simulink model "agv_mechanical_plant"  (R2026a)
settings: Solver=VariableStepAuto  StopTime=cfg.simulation.stop_time
undefined symbols (not defined in the file): cfg
settings Model: Creator=YASHRK  LastModifiedBy=YASHRK

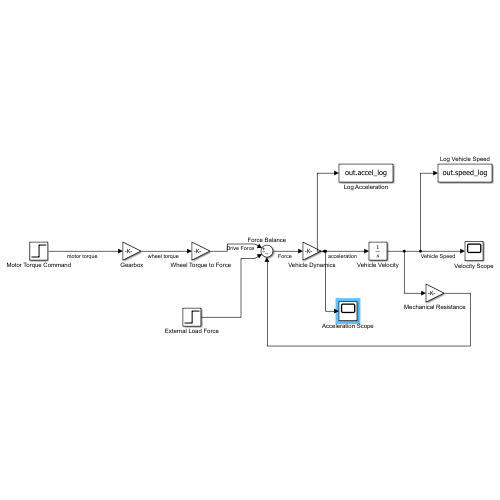
[thumbnail: Simulink's stored preview of the top-level diagram]
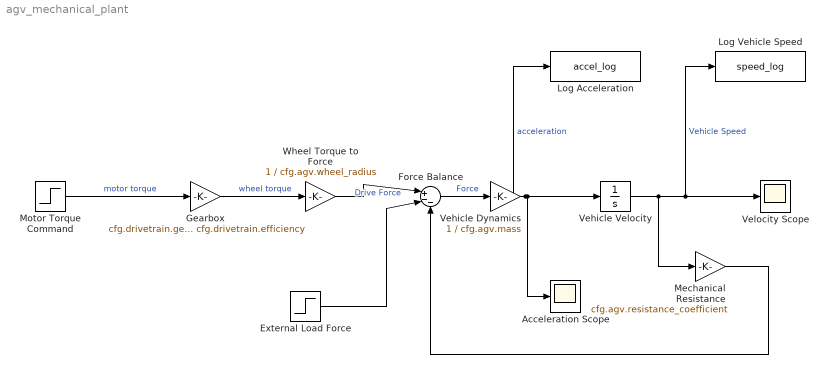
== system agv_mechanical_plant ==
  Acceleration Scope : Scope
      settings: ActiveDisplayYMinimum=-0.23749999999999996  ActiveDisplayYMaximum=2.1375
  External Load Force : Step  Time=cfg.test.phase2.load_step_time  FinalValue=cfg.test.phase2.load_force  SampleTime=0
  Force Balance : Sum  Inputs=|+--
  Gearbox : Gain  Gain=cfg.drivetrain.gear_ratio * cfg.drivetrain.efficiency
  Log Acceleration : ToWorkspace  VariableName=accel_log  SaveFormat=Timeseries  SampleTime=-1
  Log Vehicle Speed : ToWorkspace  VariableName=speed_log  SaveFormat=Timeseries  SampleTime=-1
  Mechanical Resistance : Gain  Gain=cfg.agv.resistance_coefficient
  Motor Torque Command : Step  Time=cfg.test.phase2.torque_step_time  FinalValue=cfg.test.phase2.motor_torque  SampleTime=0
  Vehicle Dynamics : Gain  Gain=1 / cfg.agv.mass
  Vehicle Velocity : Integrator
  Velocity Scope : Scope
      settings: ActiveDisplayYMinimum=-0.50967179419409014  ActiveDisplayYMaximum=4.5870461477468121
  Wheel Torque to Force : Gain  Gain=1 / cfg.agv.wheel_radius
  wires:
  Motor Torque Command/1 -> Gearbox/1  "motor torque"
  Gearbox/1 -> Wheel Torque to Force/1  "wheel torque"
  Wheel Torque to Force/1 -> Force Balance/1  "Drive Force"
  Force Balance/1 -> Vehicle Dynamics/1  "Force"
  Vehicle Dynamics/1 -> Log Acceleration/1, Acceleration Scope/1, Vehicle Velocity/1  "acceleration"
  Vehicle Velocity/1 -> Mechanical Resistance/1, Log Vehicle Speed/1, Velocity Scope/1  "Vehicle Speed"
  External Load Force/1 -> Force Balance/2
  Mechanical Resistance/1 -> Force Balance/3
